simulink library "sensors"  (R2018a)
settings: Solver=VariableStepAuto  StartTime=0.0  StopTime=10.0  RelTol=1e-3
undefined symbols (not defined in the file): magnitude
libraries: simulink_extras x10
settings Model: Creator=David  LastModifiedBy=David

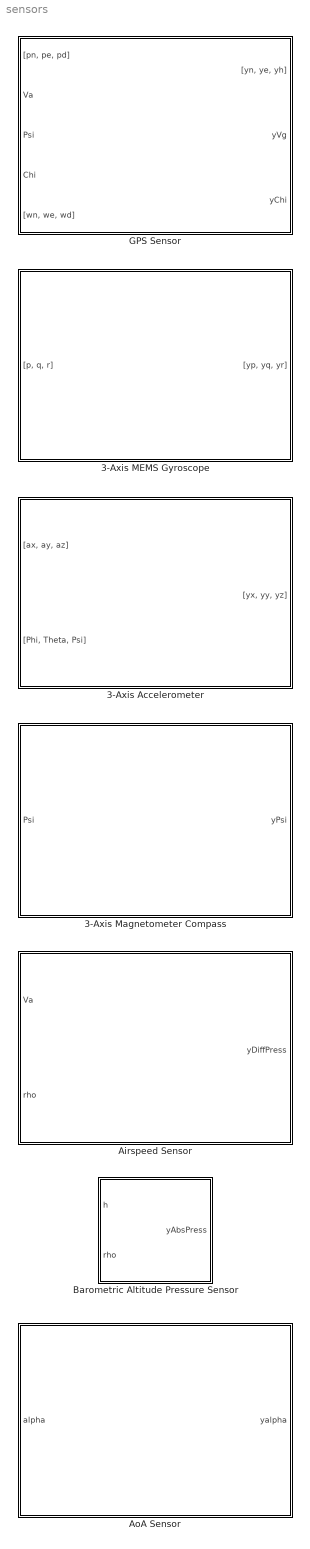
== system sensors ==
  3-Axis Accelerometer : Subsystem  mask{g=9.81, SampleTime=0.01, accelXNoiseDensity=0.1/sqrt(100), accelYNoiseDensity=0.1/sqrt(100), accelZNoiseDensity=0.1/sqrt(100), accelXBandwidthHz=1000, accelYBandwidthHz=1000, accelZBandwidthHz=1000, accelXInit=0, accelYInit=0, accelZInit=0, accelXUpperSaturation=inf, accelXLowerSaturation=-inf, accelYUpperSaturation=inf, accelYLowerSaturation=-inf, accelZUpperSaturation=inf, accelZLowerSaturation=-inf, accelXResolution=1E-12, accelYResolution=1E-12, accelZResolution=1E-12}
      mask prompts: g "Gravity (m/s^2)"; SampleTime "Accelerometer Sample Time (s)"; accelXNoiseDensity "X Accelerometer Noise Density (m/s^2/sqrt(Hz))"; accelYNoiseDensity "Y Accelerometer Noise Density (m/s^2/sqrt(Hz))"; accelZNoiseDensity "Z Accelerometer Noise Density (m/s^2/sqrt(Hz))"; accelXBandwidthHz "X Accelerometer Bandwidth (Hz)"; accelYBandwidthHz "Y Accelerometer Bandwidth (Hz)"; accelZBandwidthHz "Z Accelerometer Bandwidth (Hz)"; accelXInit "X Accelerometer Initial Condition (m/s^2)"; accelYInit "Y Accelerometer Initial Condition (m/s^2)"; accelZInit "Z Accelerometer Initial Condition (m/s^2)"; accelXUpperSaturation "X Accelerometer Measurement Upper Saturation Limit (m/s^2)"; accelXLowerSaturation "X Accelerometer Measurement Lower Saturation Limit (m/s^2)"; accelYUpperSaturation "Y Accelerometer Measurement Upper Saturation Limit (m/s^2)"; accelYLowerSaturation "Y Accelerometer Measurement Lower Saturation Limit (m/s^2)"; accelZUpperSaturation "Z Accelerometer Measurement Upper Saturation Limit (m/s^2)"; accelZLowerSaturation "Z Accelerometer Measurement Upper Saturation Limit (m/s^2)"; accelXResolution "X Accelerometer Resolution (m/s^2)"; accelYResolution "Y Accelerometer Resolution (m/s^2)"; accelZResolution "Z Accelerometer Resolution (m/s^2)"
      mask DialogControl DescGroupVar Prompt: MEMS Accelerometer Model
      mask DialogControl DescTextVar Prompt: MEMS Accelerometer Model with White Noise Modelling
      mask DialogControl Container7 Prompt: System Characteristics
      mask DialogControl Container4 Prompt: Noise Characteristics
      mask DialogControl Container8 Prompt: Density
      mask DialogControl Container10 Prompt: Sensor Dynamics
      mask DialogControl Container13 Prompt: Bandwidth
      mask DialogControl Container12 Prompt: Initial Conditions
      mask DialogControl Container15 Prompt: Limits and Quantization
      mask DialogControl Container17 Prompt: Limits
      mask DialogControl Container20 Prompt: Quantization
      mask DialogControl Control2 Prompt: This can be calculated with the following equation:
      mask DialogControl Control3 Prompt: Physical Resolution = measurement_span/(2^resolution_bits - 1)
      mask Display:
      | image('mems_accel.png')
      | 
      | color('red')
      | 
      | port_label('input', 1, '[a_x, a_y, a_z] (m/s^2)', 'texMode', 'on')
      | port_label('input', 2, '[\phi, \theta, \psi] (rad)', 'texMode', 'on')
      | 
      | port_label('output', 1, '[y_{accel_x}, y_{accel_y}, y_{accel_z}] (m/s^2)', 'texMode', 'on')
  3-Axis MEMS Gyroscope : Subsystem  mask{SampleTime=0.01, gyroXNoiseDensity=0, gyroYNoiseDensity=0, gyroZNoiseDensity=0, gyroXBandwidthHz=1E06, gyroYBandwidthHz=1E06, gyroZBandwidthHz=1E06, gyroXInit=0, gyroYInit=0, gyroZInit=0, gyroXUpperSaturation=inf, gyroXLowerSaturation=-inf, gyroYUpperSaturation=inf, gyroYLowerSaturation=-inf, gyroZUpperSaturation=inf, gyroZLowerSaturation=-inf, gyroXResolution=1E-06, gyroYResolution=1E-06, gyroZResolution=1E-06}
      mask prompts: SampleTime "Gyroscope Sample Time (s)"; gyroXNoiseDensity "X Gyroscope Noise Density (rad/s/sqrt(Hz))"; gyroYNoiseDensity "Y Gyroscope Noise Density (rad/s/sqrt(Hz))"; gyroZNoiseDensity "Z Gyroscope Noise Density (rad/s/sqrt(Hz))"; gyroXBandwidthHz "X Gyroscope Bandwidth (Hz)"; gyroYBandwidthHz "Y Gyroscope Bandwidth (Hz)"; gyroZBandwidthHz "Z Gyroscope Bandwidth (Hz)"; gyroXInit "X Gyroscope Initial Condition (rad/s)"; gyroYInit "Y Gyroscope Initial Condition (rad/s)"; gyroZInit "Z Gyroscope Initial Condition (rad/s)"; gyroXUpperSaturation "X Gyroscope Measurement Upper Saturation Limit (rad/s)"; gyroXLowerSaturation "X Gyroscope Measurement Lower Saturation Limit (rad/s)"; gyroYUpperSaturation "Y Gyroscope Measurement Upper Saturation Limit (rad/s)"; gyroYLowerSaturation "Y Gyroscope Measurement Lower Saturation Limit (rad/s)"; gyroZUpperSaturation "Z Gyroscope Measurement Upper Saturation Limit (rad/s)"; gyroZLowerSaturation "Z Gyroscope Measurement Lower Saturation Limit (rad/s)"; gyroXResolution "X Gyroscope Resolution (rad/s)"; gyroYResolution "Y Gyroscope Resolution (rad/s)"; gyroZResolution "Z Gyroscope Resolution (rad/s)"
      mask DialogControl DescGroupVar Prompt: MEMS Gyroscope Model
      mask DialogControl DescTextVar Prompt: MEMS Gyroscope Model with White Noise Modelling
      mask DialogControl Container7 Prompt: System Characteristics
      mask DialogControl Container4 Prompt: Noise Characteristics
      mask DialogControl Container6 Prompt: Sensor Dynamics
      mask DialogControl Container9 Prompt: Bandwidth
      mask DialogControl Container10 Prompt: Initial Conditions
      mask DialogControl Container11 Prompt: Limits and Quantization
      mask DialogControl Container13 Prompt: Limits
      mask DialogControl Container14 Prompt: Quantization
      mask DialogControl Control3 Prompt: This can be calculated with the following equation:
      mask DialogControl Control2 Prompt: Physical Resolution = measurement_span/(2^resolution_bits - 1)
      mask Display:
      | image('mems_gyro.jpg')
      | 
      | color('red')
      | 
      | port_label('input', 1, '[p, q, r] (rad/s)', 'texMode', 'on')
      | 
      | port_label('output', 1, '[y_{gyro_p}, y_{gyro_q}, y_{gyro_r}] (rad/s)', 'texMode', 'on')
  3-Axis Magnetometer Compass : Subsystem  mask{SampleTime=1, headingNoiseDensity=0, headingBandwidthHz=1E06, headingInit=0, headingUpperSaturation=inf, headingLowerSaturation=-inf, headingResolution=1E-06}
      mask prompts: SampleTime "Magnetometer Sample Time (s)"; headingNoiseDensity "Magnetometer Heading Noise Density (rad/sqrt(Hz))"; headingBandwidthHz "Magnetometer Heading Sensor Bandwidth (Hz)"; headingInit "Magnetometer Heading Sensor Initial Condition (rad)"; headingUpperSaturation "Magnetometer Heading Sensor Upper Saturation Limit (rad)"; headingLowerSaturation "Magnetometer Heading Sensor Lower Saturation Limit (rad)"; headingResolution "Magnetometer Heading Sensor Resolution (rad)"
      mask DialogControl DescGroupVar Prompt: MEMS Magnetometer Model
      mask DialogControl DescTextVar Prompt: MEMS Magnetometer Model to Estimate Heading Angle with White Noise Modelling
      mask DialogControl Container7 Prompt: System Characteristics
      mask DialogControl Container4 Prompt: Noise Characteristics
      mask DialogControl Container6 Prompt: Sensor Dynamics
      mask DialogControl Container10 Prompt: Bandwidth
      mask DialogControl Container11 Prompt: Initial Conditions
      mask DialogControl Container8 Prompt: Limits and Quantization
      mask DialogControl Container13 Prompt: Limits
      mask DialogControl Container14 Prompt: Quantization
      mask Display:
      | image('mems_compass.jpg')
      | 
      | color('red')
      | 
      | port_label('input', 1, '\psi (rad)', 'texMode', 'on')
      | 
      | port_label('output', 1, 'y_{\psi} (rad)', 'texMode', 'on')
  Airspeed Sensor : Subsystem  mask{SampleTime=1, diffPressureStdDev=0, diffPressureBandwidthHz=1E06, diffPressureInit=0, diffPressureUpperSaturation=inf, diffPressureLowerSaturation=-inf, diffPressureResolution=1E-12}
      mask prompts: SampleTime "Airspeed Sensor Sample Time (s)"; diffPressureStdDev "Airspeed Pressure Sensor Noise Std Dev (Pa)"; diffPressureBandwidthHz "Airspeed Pressure Sensor Bandwidth (Hz)"; diffPressureInit "Airspeed Pressure Sensor Initial Condition (Pa)"; diffPressureUpperSaturation "Airspeed Pressure Sensor Upper Saturation Limit (Pa)"; diffPressureLowerSaturation "Airspeed Pressure Sensor Lower Saturation Limit (Pa)"; diffPressureResolution "Airspeed Pressure Sensor Resolution (Pa)"
      mask DialogControl DescGroupVar Prompt: Pitot Tube Airspeed Sensor Model
      mask DialogControl DescTextVar Prompt: Pitot Tube Airspeed Sensor with White Noise Modelling.
      mask DialogControl Control2 Prompt: If one can only get a sensor accuracy of +- error band of span, treat this as 4 sigma when calculating noise density (8 sigma ~ peak-to-peak). (ie. std dev = ((Sensor % Band)/4)*Span )
      mask DialogControl Container7 Prompt: System Characteristics
      mask DialogControl Container4 Prompt: Noise Characteristics
      mask DialogControl Container6 Prompt: Sensor Dynamics
      mask DialogControl Container10 Prompt: Bandwidth
      mask DialogControl Container11 Prompt: Initial Conditions
      mask DialogControl Container8 Prompt: Limits and Quantization
      mask DialogControl Container13 Prompt: Limits
      mask DialogControl Container16 Prompt: Quantization
      mask Display:
      | image('airspeed_sensor.jpg')
      | 
      | color('green')
      | 
      | port_label('input', 1, 'V_a (m/s)', 'texMode', 'on')
      | port_label('input', 2, '\rho (kg/m^3)', 'texMode', 'on')
      | 
      | port_label('output', 1, 'y_{\DeltaP_{V_a}} (Pa)', 'texMode', 'on')
  AoA Sensor : Subsystem  mask{SampleTime=1, alphaStdDev=0, alphaBandwidthHz=1E06, alphaInit=0, alphaUpperSaturation=inf, alphaLowerSaturation=-inf, alphaResolution=1E-12}
      mask prompts: SampleTime "AoA Sensor Sample Time (s)"; alphaStdDev "AoA Sensor Noise Std Dev (rad)"; alphaBandwidthHz "AoA Sensor Bandwidth (Hz)"; alphaInit "AoA Sensor Initial Condition (rad)"; alphaUpperSaturation "AoA Sensor Upper Saturation Limit (rad)"; alphaLowerSaturation "AoA Sensor Lower Saturation Limit (rad)"; alphaResolution "AoA Sensor Resolution (rad)"
      mask DialogControl DescGroupVar Prompt: Pitot Tube Airspeed Sensor Model
      mask DialogControl DescTextVar Prompt: Angle of attack (alpha/AoA) sensor with White Noise Modelling.
      mask DialogControl Container7 Prompt: System Characteristics
      mask DialogControl Container4 Prompt: Noise Characteristics
      mask DialogControl Container6 Prompt: Sensor Dynamics
      mask DialogControl Container10 Prompt: Bandwidth
      mask DialogControl Container11 Prompt: Initial Conditions
      mask DialogControl Container8 Prompt: Limits and Quantization
      mask DialogControl Container13 Prompt: Limits
      mask DialogControl Container16 Prompt: Quantization
      mask Display:
      | image('aoa_sensor.png')
      | 
      | color('green')
      | 
      | port_label('input', 1, '\alpha (rad)', 'texMode', 'on')
      | 
      | port_label('output', 1, 'y_{\alpha} (rad)', 'texMode', 'on')
  Barometric Altitude Pressure Sensor : Subsystem  mask{g=9.81, SampleTime=1, absPressureStdDev=0, absPressureBandwidthHz=1E06, absPressureInit=0, absPressureUpperSaturation=inf, absPressureLowerSaturation=-inf, absPressureResolution=1E-12}
      mask prompts: g "Gravity (m/s^2)"; SampleTime "Barometric Altitude Pressure Sensor Sample Time (s)"; absPressureStdDev "Barometric Altitude Pressure Sensor Noise Std Dev (Pa)"; absPressureBandwidthHz "Barometric Altitude Pressure Sensor Bandwidth (Hz)"; absPressureInit "Barometric Altitude Pressure Sensor Initial Condition (Pa)"; absPressureUpperSaturation "Barometric Altitude Sensor Upper Saturation Limit (Pa)"; absPressureLowerSaturation "Barometric Altitude Sensor Lower Saturation Limit (Pa)"; absPressureResolution "Barometric Altitude Pressure Sensor Resolution (Pa)"
      mask DialogControl DescGroupVar Prompt: Barometric Altitude Pressure Sensor Model
      mask DialogControl DescTextVar Prompt: Barometric Altitude Pressure Sensor with White Noise Modelling.
      mask DialogControl Control2 Prompt: If one can only get a sensor accuracy of +- error band of span, treat this as 4 sigma when calculating noise density (8 sigma ~ peak-to-peak). (ie. std dev = ((Sensor % Band)/4)*Span )
      mask DialogControl Container7 Prompt: System Characteristics
      mask DialogControl Container4 Prompt: Noise Characteristics
      mask DialogControl Container6 Prompt: Sensor Dynamics
      mask DialogControl Container10 Prompt: Bandwidth
      mask DialogControl Container11 Prompt: Initial Conditions
      mask DialogControl Container8 Prompt: Limits and Quantization
      mask DialogControl Container13 Prompt: Limits
      mask DialogControl Container16 Prompt: Quantization
      mask Display:
      | image('barometer.jpg')
      | 
      | color('green')
      | 
      | port_label('input', 1, 'h (m)', 'texMode', 'on')
      | port_label('input', 2, '\rho (kg/m^3)', 'texMode', 'on')
      | 
      | port_label('output', 1, 'y_{P_{abs}} (Pa)', 'texMode', 'on')
  GPS Sensor : Subsystem  mask{SampleTime=0.2, pnInit=0, peInit=0, pdInit=0, VgInit=0, ChiInit=0, GPSNStdDev=0.21, OneOverkGPSN=1100, GPSEStdDev=0.21, OneOverkGPSE=1100, GPSAltStdDev=0.4, OneOverkGPSAlt=1100, GPSVStdDev=0.2}
      mask prompts: SampleTime "GPS Sample Time (s)"; pnInit "Initial North Position (m)"; peInit "Initial East Position (m)"; pdInit "Initial Down Position (m) (-altitude)"; VgInit "Initial Vg (m/s)"; ChiInit "Initial Chi (rad)"; GPSNStdDev "GPS North Std Dev (m)"; OneOverkGPSN "GPS North Time Constant (s)"; GPSEStdDev "GPS East Std Dev (m)"; OneOverkGPSE "GPS East Time Constant (s)"; GPSAltStdDev "GPS Altitude Std Dev (m)"; OneOverkGPSAlt "GPS Altitude Time Constant (s)"; GPSVStdDev "GPS Velocity Std Dev (m/s)"
      mask DialogControl DescGroupVar Prompt: GPS Sensor Model
      mask DialogControl DescTextVar Prompt: GPS Sensor Model Making use of a Gauss-Markov process for noise modelling
      mask DialogControl Container4 Prompt: System Characteristics
      mask DialogControl Container5 Prompt: Noise Characteristics
      mask Display:
      | image('PiksiMulti_GPS.jpg')
      | 
      | color('green')
      | 
      | port_label('input', 1, '[p_N, p_E, p_D] (m)', 'texMode', 'On')
      | port_label('input', 2, 'V_a (m/s)', 'texMode', 'On')
      | port_label('input', 3, '\psi (rad)', 'texMode', 'On')
      | port_label('input', 4, '\chi (rad)', 'texMode', 'On')
      | port_label('input', 5, '[w_N, w_E, w_D] (m/s)', 'texMode', 'On')
      | 
      | port_label('output', 1, '[y_{GPS_N}, y_{GPS_E}, y_{GPS_h}] (m)', 'texMode', 'On')
      | port_label('output', 2, 'y_{GPS_{Vg}} (m/s)', 'texMode', 'On')
      | port_label('output', 3, 'y_{GPS_{\chi}} (rad)', 'texMode', 'On')

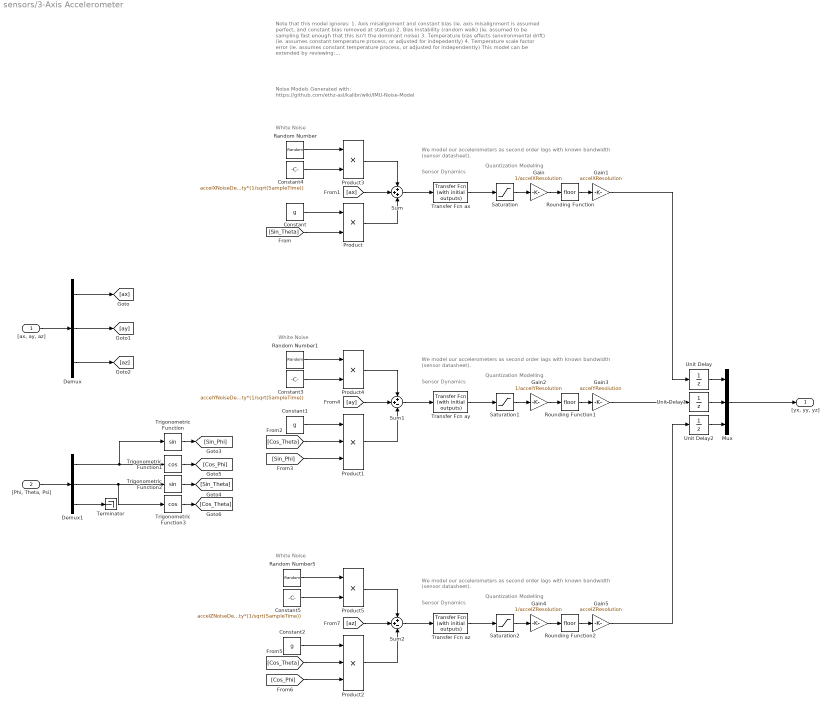
== system sensors/3-Axis Accelerometer ==
  note: Quantization Modelling
  note: Sensor Dynamics
  note: Note that this model ignores:
      | 1. Axis misalignment and constant bias (ie. axis misalignment is assumed perfect, and constant bias removed at startup)
      | 2. Bias Instability (random walk) (ie. assumed to be sampling fast enough that this isn't the dominant noise)
      | 3. Temperature bias effects (environmental drift) (ie. assumes constant temperature process, or adjusted for indepedently)
      | 4. Temperature scale factor error (ie. assumes constant temperature process, or adjusted for independently)
      |
      | This model can be extended by reviewing:
      | https://www.mathworks.com/help/fusion/ref/imusensor-system-object.html?searchHighlight=imuSensor&s_tid=doc_srchtitle
  note: We model our accelerometers as second order lags with known bandwidth
      | (sensor datasheet).
  note: White Noise
  note: Noise Models Generated with:
      | https://github.com/ethz-asl/kalibr/wiki/IMU-Noise-Model
  note: White Noise
  note: White Noise
  note: We model our accelerometers as second order lags with known bandwidth
      | (sensor datasheet).
  note: Quantization Modelling
  note: Sensor Dynamics
  note: We model our accelerometers as second order lags with known bandwidth
      | (sensor datasheet).
  note: Quantization Modelling
  note: Sensor Dynamics
  "[ax, ay, az]" : Inport
  "[Phi, Theta, Psi]" : Inport  Port=2
  Constant : Constant  Value=g
  Constant1 : Constant  Value=g
  Constant2 : Constant  Value=g
  Constant3 : Constant  Value=accelYNoiseDensity*(1/sqrt(SampleTime))
  Constant4 : Constant  Value=accelXNoiseDensity*(1/sqrt(SampleTime))
  Constant5 : Constant  Value=accelZNoiseDensity*(1/sqrt(SampleTime))
  Demux : Demux  Outputs=3
  Demux1 : Demux  Outputs=3
  Gain : Gain  Gain=1/accelXResolution
  Gain1 : Gain  Gain=accelXResolution
  Gain2 : Gain  Gain=1/accelYResolution
  Gain3 : Gain  Gain=accelYResolution
  Gain4 : Gain  Gain=1/accelZResolution
  Gain5 : Gain  Gain=accelZResolution
  Mux : Mux  Inputs=3
  Product{,3..5} (4 alike) : Product
  Product1 : Product  Inputs=3
  Product2 : Product  Inputs=3
  Random Number : RandomNumber  SampleTime=SampleTime
  Random Number1 : RandomNumber  SampleTime=SampleTime
  Random Number5 : RandomNumber  SampleTime=SampleTime
  Rounding Function : Rounding
  Rounding Function1 : Rounding
  Rounding Function2 : Rounding
  Saturation : Saturate  UpperLimit=accelXUpperSaturation  LowerLimit=accelXLowerSaturation  ZeroCross=off
  Saturation1 : Saturate  UpperLimit=accelYUpperSaturation  LowerLimit=accelYLowerSaturation  ZeroCross=off
  Saturation2 : Saturate  UpperLimit=accelZUpperSaturation  LowerLimit=accelZLowerSaturation  ZeroCross=off
  Sum : Sum  Inputs=+++
  Sum1 : Sum  Inputs=++-
  Sum2 : Sum  Inputs=++-
  Terminator : Terminator
  Transfer Fcn ax : simulink_extras/Additional Linear/Transfer Fcn (with initial outputs)  N=[(accelXBandwidthHz*2*pi)^2]  D="[1,  2*accelXBandwidthHz*2*pi, (accelXBandwidthHz*2*pi)^2]"  Y0=accelXInit  U0=accelXInit
  Transfer Fcn ay : simulink_extras/Additional Linear/Transfer Fcn (with initial outputs)  N=[(accelYBandwidthHz*2*pi)^2]  D="[1,  2*accelYBandwidthHz*2*pi, (accelYBandwidthHz*2*pi)^2]"  Y0=accelXInit  U0=accelXInit
  Transfer Fcn az : simulink_extras/Additional Linear/Transfer Fcn (with initial outputs)  N=[(accelZBandwidthHz*2*pi)^2]  D="[1,  2*accelZBandwidthHz*2*pi, (accelZBandwidthHz*2*pi)^2]"  Y0=accelXInit  U0=accelXInit
  Trigonometric Function : Trigonometry
  Trigonometric Function1 : Trigonometry  Operator=cos
  Trigonometric Function2 : Trigonometry
  Trigonometric Function3 : Trigonometry  Operator=cos
  Unit Delay : UnitDelay  InitialCondition=accelXInit  SampleTime=SampleTime
  Unit Delay1 : UnitDelay  InitialCondition=accelYInit  SampleTime=SampleTime
  Unit Delay2 : UnitDelay  InitialCondition=accelZInit  SampleTime=SampleTime
  "[yx, yy, yz]" : Outport
  wires:
  Product/1 -> Sum/3
  [ax] -> Sum/2
  Trigonometric Function3/1 -> [Cos_Theta]
  Sum/1 -> Transfer Fcn ax/1
  Mux/1 -> "[yx, yy, yz]"/1
  [Cos_Phi] -> Product2/3
  Trigonometric Function2/1 -> [Sin_Theta]
  Constant2/1 -> Product2/1
  Demux1/1 -> Trigonometric Function1/1, Trigonometric Function/1
  Demux1/2 -> Trigonometric Function3/1, Trigonometric Function2/1
  [Sin_Theta] -> Product/2
  "[Phi, Theta, Psi]"/1 -> Demux1/1
  [Cos_Theta] -> Product2/2
  [az] -> Sum2/2
  [Cos_Theta] -> Product1/2
  Product2/1 -> Sum2/3
  Trigonometric Function/1 -> [Sin_Phi]
  [ay] -> Sum1/2
  Product1/1 -> Sum1/3
  [Sin_Phi] -> Product1/3
  Trigonometric Function1/1 -> [Cos_Phi]
  Constant1/1 -> Product1/1
  Constant/1 -> Product/1
  Demux1/3 -> Terminator/1
  "[ax, ay, az]"/1 -> Demux/1
  Random Number/1 -> Product3/1
  Constant4/1 -> Product3/2
  Constant3/1 -> Product4/2
  Constant5/1 -> Product5/2
  Demux/1 -> [ax]
  Demux/2 -> [ay]
  Demux/3 -> [az]
  Product3/1 -> Sum/1
  Product4/1 -> Sum1/1
  Random Number1/1 -> Product4/1
  Random Number5/1 -> Product5/1
  Product5/1 -> Sum2/1
  Saturation/1 -> Gain/1
  Transfer Fcn ax/1 -> Saturation/1
  Gain/1 -> Rounding Function/1
  Rounding Function/1 -> Gain1/1
  Gain1/1 -> Unit Delay/1
  Gain2/1 -> Rounding Function1/1
  Saturation1/1 -> Gain2/1
  Transfer Fcn ay/1 -> Saturation1/1
  Rounding Function1/1 -> Gain3/1
  Sum1/1 -> Transfer Fcn ay/1
  Gain3/1 -> Unit Delay1/1
  Gain5/1 -> Unit Delay2/1
  Sum2/1 -> Transfer Fcn az/1
  Rounding Function2/1 -> Gain5/1
  Saturation2/1 -> Gain4/1
  Transfer Fcn az/1 -> Saturation2/1
  Gain4/1 -> Rounding Function2/1
  Unit Delay/1 -> Mux/1
  Unit Delay1/1 -> Mux/2
  Unit Delay2/1 -> Mux/3

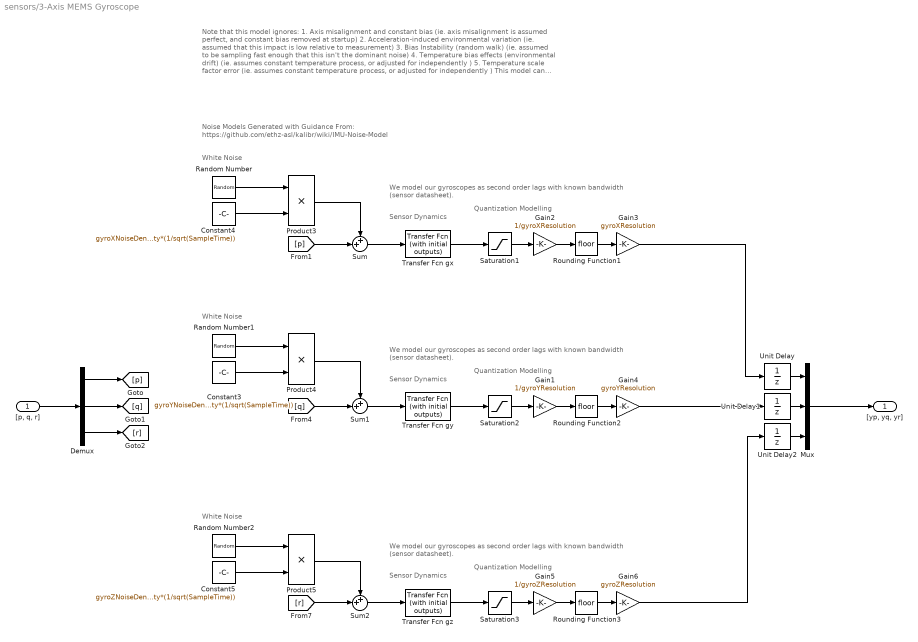
== system sensors/3-Axis MEMS Gyroscope ==
  note: White Noise
  note: Noise Models Generated with Guidance From:
      | https://github.com/ethz-asl/kalibr/wiki/IMU-Noise-Model
  note: White Noise
  note: White Noise
  note: We model our gyroscopes as second order lags with known bandwidth
      | (sensor datasheet).
  note: Quantization Modelling
  note: Sensor Dynamics
  note: Quantization Modelling
  note: Sensor Dynamics
  note: We model our gyroscopes as second order lags with known bandwidth
      | (sensor datasheet).
  note: Quantization Modelling
  note: We model our gyroscopes as second order lags with known bandwidth
      | (sensor datasheet).
  note: Sensor Dynamics
  note: Note that this model ignores:
      | 1. Axis misalignment and constant bias (ie. axis misalignment is assumed perfect, and constant bias removed at startup)
      | 2. Acceleration-induced environmental variation (ie. assumed that this impact is low relative to measurement)
      | 3. Bias Instability (random walk) (ie. assumed to be sampling fast enough that this isn't the dominant noise)
      | 4. Temperature bias effects (environmental drift) (ie. assumes constant temperature process, or adjusted for independently )
      | 5. Temperature scale factor error (ie. assumes constant temperature process, or adjusted for independently )
      |
      | This model can be extended by reviewing:
      | https://www.mathworks.com/help/fusion/ref/imusensor-system-object.html?searchHighlight=imuSensor&s_tid=doc_srchtitle
  "[p, q, r]" : Inport
  Constant3 : Constant  Value=gyroYNoiseDensity*(1/sqrt(SampleTime))
  Constant4 : Constant  Value=gyroXNoiseDensity*(1/sqrt(SampleTime))
  Constant5 : Constant  Value=gyroZNoiseDensity*(1/sqrt(SampleTime))
  Demux : Demux  Outputs=3
  Gain1 : Gain  Gain=1/gyroYResolution
  Gain2 : Gain  Gain=1/gyroXResolution
  Gain3 : Gain  Gain=gyroXResolution
  Gain4 : Gain  Gain=gyroYResolution
  Gain5 : Gain  Gain=1/gyroZResolution
  Gain6 : Gain  Gain=gyroZResolution
  Mux : Mux  Inputs=3
  Product3 : Product
  Product4 : Product
  Product5 : Product
  Random Number : RandomNumber  SampleTime=SampleTime
  Random Number1 : RandomNumber  SampleTime=SampleTime
  Random Number2 : RandomNumber  SampleTime=SampleTime
  Rounding Function1 : Rounding
  Rounding Function2 : Rounding
  Rounding Function3 : Rounding
  Saturation1 : Saturate  UpperLimit=gyroXUpperSaturation  LowerLimit=gyroXLowerSaturation
  Saturation2 : Saturate  UpperLimit=gyroYUpperSaturation  LowerLimit=gyroYLowerSaturation
  Saturation3 : Saturate  UpperLimit=gyroZUpperSaturation  LowerLimit=gyroZLowerSaturation
  Sum : Sum  Inputs=++|
  Sum1 : Sum  Inputs=++|
  Sum2 : Sum  Inputs=++|
  Transfer Fcn gx : simulink_extras/Additional Linear/Transfer Fcn (with initial outputs)  N=[(gyroXBandwidthHz*2*pi)^2]  D="[1,  2*gyroXBandwidthHz*2*pi, (gyroXBandwidthHz*2*pi)^2]"  Y0=gyroXInit  U0=gyroXInit
  Transfer Fcn gy : simulink_extras/Additional Linear/Transfer Fcn (with initial outputs)  N=[(gyroYBandwidthHz*2*pi)^2]  D="[1,  2*gyroYBandwidthHz*2*pi, (gyroYBandwidthHz*2*pi)^2]"  Y0=gyroYInit  U0=gyroYInit
  Transfer Fcn gz : simulink_extras/Additional Linear/Transfer Fcn (with initial outputs)  N=[(gyroZBandwidthHz*2*pi)^2]  D="[1,  2*gyroZBandwidthHz*2*pi, (gyroZBandwidthHz*2*pi)^2]"  Y0=gyroZInit  U0=gyroZInit
  Unit Delay : UnitDelay  InitialCondition=gyroXInit  SampleTime=SampleTime
  Unit Delay1 : UnitDelay  InitialCondition=gyroYInit  SampleTime=SampleTime
  Unit Delay2 : UnitDelay  InitialCondition=gyroZInit  SampleTime=SampleTime
  "[yp, yq, yr]" : Outport
  wires:
  [p] -> Sum/2
  Demux/3 -> [r]
  Mux/1 -> "[yp, yq, yr]"/1
  [r] -> Sum2/2
  [q] -> Sum1/2
  Demux/1 -> [p]
  Demux/2 -> [q]
  "[p, q, r]"/1 -> Demux/1
  Random Number/1 -> Product3/1
  Product3/1 -> Sum/1
  Constant4/1 -> Product3/2
  Random Number1/1 -> Product4/1
  Constant3/1 -> Product4/2
  Product4/1 -> Sum1/1
  Product5/1 -> Sum2/1
  Constant5/1 -> Product5/2
  Random Number2/1 -> Product5/1
  Gain3/1 -> Unit Delay/1
  Sum/1 -> Transfer Fcn gx/1
  Rounding Function1/1 -> Gain3/1
  Saturation1/1 -> Gain2/1
  Transfer Fcn gx/1 -> Saturation1/1
  Gain2/1 -> Rounding Function1/1
  Saturation2/1 -> Gain1/1
  Sum1/1 -> Transfer Fcn gy/1
  Gain4/1 -> Unit Delay1/1
  Rounding Function2/1 -> Gain4/1
  Gain1/1 -> Rounding Function2/1
  Transfer Fcn gy/1 -> Saturation2/1
  Sum2/1 -> Transfer Fcn gz/1
  Gain5/1 -> Rounding Function3/1
  Rounding Function3/1 -> Gain6/1
  Transfer Fcn gz/1 -> Saturation3/1
  Saturation3/1 -> Gain5/1
  Gain6/1 -> Unit Delay2/1
  Unit Delay/1 -> Mux/1
  Unit Delay1/1 -> Mux/2
  Unit Delay2/1 -> Mux/3

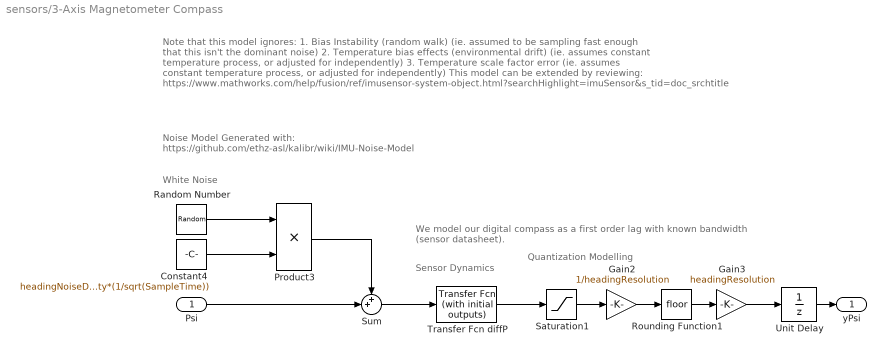
== system sensors/3-Axis Magnetometer Compass ==
  note: White Noise
  note: Noise Model Generated with:
      | https://github.com/ethz-asl/kalibr/wiki/IMU-Noise-Model
  note: Quantization Modelling
  note: We model our digital compass as a first order lag with known bandwidth
      | (sensor datasheet).
  note: Sensor Dynamics
  note: Note that this model ignores:
      | 1. Bias Instability (random walk) (ie. assumed to be sampling fast enough that this isn't the dominant noise)
      | 2. Temperature bias effects (environmental drift) (ie. assumes constant temperature process, or adjusted for independently)
      | 3. Temperature scale factor error (ie. assumes constant temperature process, or adjusted for independently)
      |
      | This model can be extended by reviewing:
      | https://www.mathworks.com/help/fusion/ref/imusensor-system-object.html?searchHighlight=imuSensor&s_tid=doc_srchtitle
  Psi : Inport
  Constant4 : Constant  Value=headingNoiseDensity*(1/sqrt(SampleTime))
  Gain2 : Gain  Gain=1/headingResolution
  Gain3 : Gain  Gain=headingResolution
  Product3 : Product
  Random Number : RandomNumber  SampleTime=SampleTime
  Rounding Function1 : Rounding
  Saturation1 : Saturate  UpperLimit=headingUpperSaturation  LowerLimit=headingLowerSaturation
  Sum : Sum  Inputs=++|
  Transfer Fcn diffP : simulink_extras/Additional Linear/Transfer Fcn (with initial outputs)  N=[headingBandwidthHz*2*pi]  D="[1,  headingBandwidthHz*2*pi]"  Y0=headingInit  U0=headingInit
  Unit Delay : UnitDelay  InitialCondition=headingInit  SampleTime=SampleTime
  yPsi : Outport
  wires:
  Psi/1 -> Sum/2
  Random Number/1 -> Product3/1
  Product3/1 -> Sum/1
  Constant4/1 -> Product3/2
  Sum/1 -> Transfer Fcn diffP/1
  Rounding Function1/1 -> Gain3/1
  Gain2/1 -> Rounding Function1/1
  Saturation1/1 -> Gain2/1
  Transfer Fcn diffP/1 -> Saturation1/1
  Gain3/1 -> Unit Delay/1
  Unit Delay/1 -> yPsi/1

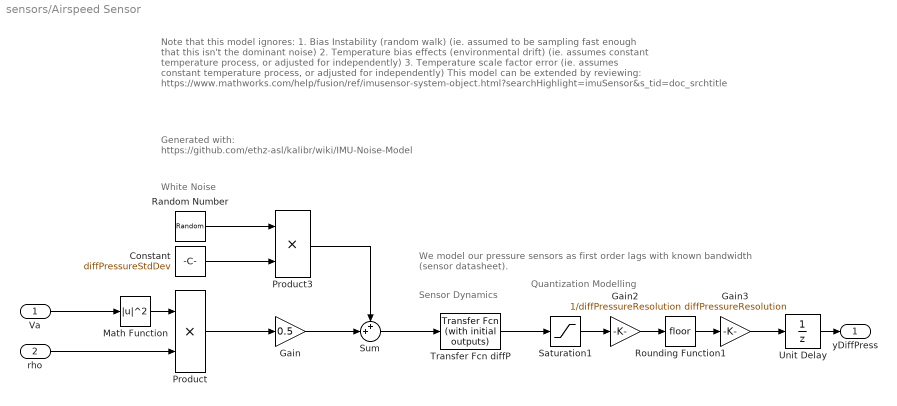
== system sensors/Airspeed Sensor ==
  note: White Noise
  note: Generated with:
      | https://github.com/ethz-asl/kalibr/wiki/IMU-Noise-Model
  note: We model our pressure sensors as first order lags with known bandwidth
      | (sensor datasheet).
  note: Sensor Dynamics
  note: Quantization Modelling
  note: Note that this model ignores:
      | 1. Bias Instability (random walk) (ie. assumed to be sampling fast enough that this isn't the dominant noise)
      | 2. Temperature bias effects (environmental drift) (ie. assumes constant temperature process, or adjusted for independently)
      | 3. Temperature scale factor error (ie. assumes constant temperature process, or adjusted for independently)
      |
      | This model can be extended by reviewing:
      | https://www.mathworks.com/help/fusion/ref/imusensor-system-object.html?searchHighlight=imuSensor&s_tid=doc_srchtitle
  Va : Inport
  rho : Inport  Port=2
  Constant : Constant  Value=diffPressureStdDev
  Gain : Gain  Gain=0.5
  Gain2 : Gain  Gain=1/diffPressureResolution
  Gain3 : Gain  Gain=diffPressureResolution
  Math Function : Math  Operator=magnitude^2  SaturateOnIntegerOverflow=on
  Product : Product
  Product3 : Product
  Random Number : RandomNumber  SampleTime=SampleTime
  Rounding Function1 : Rounding
  Saturation1 : Saturate  UpperLimit=diffPressureUpperSaturation  LowerLimit=diffPressureLowerSaturation
  Sum : Sum  Inputs=++|
  Transfer Fcn diffP : simulink_extras/Additional Linear/Transfer Fcn (with initial outputs)  N=[diffPressureBandwidthHz*2*pi]  D="[1,  diffPressureBandwidthHz*2*pi]"  Y0=diffPressureInit  U0=diffPressureInit
  Unit Delay : UnitDelay  InitialCondition=diffPressureInit  SampleTime=SampleTime
  yDiffPress : Outport
  wires:
  Va/1 -> Math Function/1
  Random Number/1 -> Product3/1
  Product3/1 -> Sum/1
  Constant/1 -> Product3/2
  Math Function/1 -> Product/1
  rho/1 -> Product/2
  Product/1 -> Gain/1
  Gain/1 -> Sum/2
  Transfer Fcn diffP/1 -> Saturation1/1
  Sum/1 -> Transfer Fcn diffP/1
  Gain2/1 -> Rounding Function1/1
  Saturation1/1 -> Gain2/1
  Gain3/1 -> Unit Delay/1
  Rounding Function1/1 -> Gain3/1
  Unit Delay/1 -> yDiffPress/1

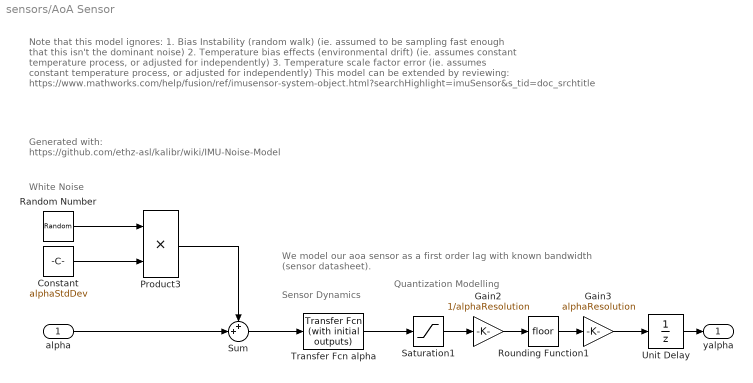
== system sensors/AoA Sensor ==
  note: White Noise
  note: Generated with:
      | https://github.com/ethz-asl/kalibr/wiki/IMU-Noise-Model
  note: We model our aoa sensor as a first order lag with known bandwidth
      | (sensor datasheet).
  note: Sensor Dynamics
  note: Quantization Modelling
  note: Note that this model ignores:
      | 1. Bias Instability (random walk) (ie. assumed to be sampling fast enough that this isn't the dominant noise)
      | 2. Temperature bias effects (environmental drift) (ie. assumes constant temperature process, or adjusted for independently)
      | 3. Temperature scale factor error (ie. assumes constant temperature process, or adjusted for independently)
      |
      | This model can be extended by reviewing:
      | https://www.mathworks.com/help/fusion/ref/imusensor-system-object.html?searchHighlight=imuSensor&s_tid=doc_srchtitle
  alpha : Inport
  Constant : Constant  Value=alphaStdDev
  Gain2 : Gain  Gain=1/alphaResolution
  Gain3 : Gain  Gain=alphaResolution
  Product3 : Product
  Random Number : RandomNumber  SampleTime=SampleTime
  Rounding Function1 : Rounding
  Saturation1 : Saturate  UpperLimit=alphaUpperSaturation  LowerLimit=alphaLowerSaturation
  Sum : Sum  Inputs=++|
  Transfer Fcn alpha : simulink_extras/Additional Linear/Transfer Fcn (with initial outputs)  N=[alphaBandwidthHz*2*pi]  D="[1,  alphaBandwidthHz*2*pi]"  Y0=alphaInit  U0=alphaInit
  Unit Delay : UnitDelay  InitialCondition=alphaInit  SampleTime=SampleTime
  yalpha : Outport
  wires:
  Random Number/1 -> Product3/1
  Product3/1 -> Sum/1
  Constant/1 -> Product3/2
  alpha/1 -> Sum/2
  Transfer Fcn alpha/1 -> Saturation1/1
  Sum/1 -> Transfer Fcn alpha/1
  Gain2/1 -> Rounding Function1/1
  Saturation1/1 -> Gain2/1
  Gain3/1 -> Unit Delay/1
  Rounding Function1/1 -> Gain3/1
  Unit Delay/1 -> yalpha/1

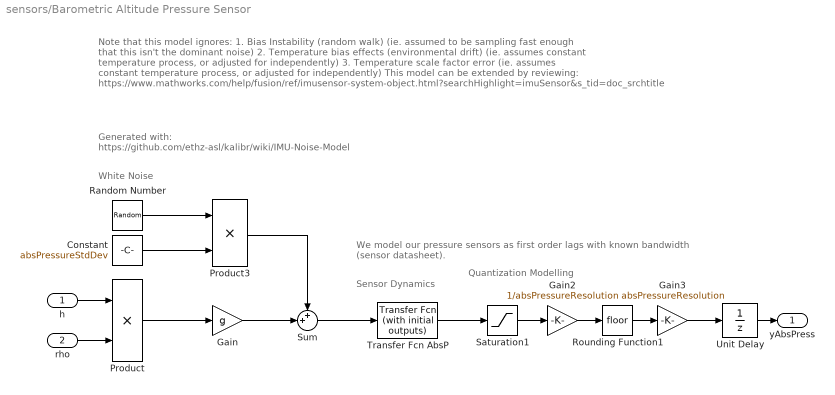
== system sensors/Barometric Altitude Pressure Sensor ==
  note: Generated with:
      | https://github.com/ethz-asl/kalibr/wiki/IMU-Noise-Model
  note: We model our pressure sensors as first order lags with known bandwidth
      | (sensor datasheet).
  note: Sensor Dynamics
  note: Quantization Modelling
  note: Note that this model ignores:
      | 1. Bias Instability (random walk) (ie. assumed to be sampling fast enough that this isn't the dominant noise)
      | 2. Temperature bias effects (environmental drift) (ie. assumes constant temperature process, or adjusted for independently)
      | 3. Temperature scale factor error (ie. assumes constant temperature process, or adjusted for independently)
      |
      | This model can be extended by reviewing:
      | https://www.mathworks.com/help/fusion/ref/imusensor-system-object.html?searchHighlight=imuSensor&s_tid=doc_srchtitle
  note: White Noise
  h : Inport
  rho : Inport  Port=2
  Constant : Constant  Value=absPressureStdDev
  Gain : Gain  Gain=g
  Gain2 : Gain  Gain=1/absPressureResolution
  Gain3 : Gain  Gain=absPressureResolution
  Product : Product
  Product3 : Product
  Random Number : RandomNumber  SampleTime=SampleTime
  Rounding Function1 : Rounding
  Saturation1 : Saturate  UpperLimit=absPressureUpperSaturation  LowerLimit=absPressureLowerSaturation
  Sum : Sum  Inputs=++|
  Transfer Fcn AbsP : simulink_extras/Additional Linear/Transfer Fcn (with initial outputs)  N=[absPressureBandwidthHz*2*pi]  D="[1,  absPressureBandwidthHz*2*pi]"  Y0=absPressureInit  U0=absPressureInit
  Unit Delay : UnitDelay  InitialCondition=absPressureInit  SampleTime=SampleTime
  yAbsPress : Outport
  wires:
  Transfer Fcn AbsP/1 -> Saturation1/1
  Sum/1 -> Transfer Fcn AbsP/1
  Gain2/1 -> Rounding Function1/1
  Saturation1/1 -> Gain2/1
  Gain3/1 -> Unit Delay/1
  Rounding Function1/1 -> Gain3/1
  Gain/1 -> Sum/2
  Constant/1 -> Product3/2
  Product3/1 -> Sum/1
  Product/1 -> Gain/1
  Random Number/1 -> Product3/1
  rho/1 -> Product/2
  h/1 -> Product/1
  Unit Delay/1 -> yAbsPress/1

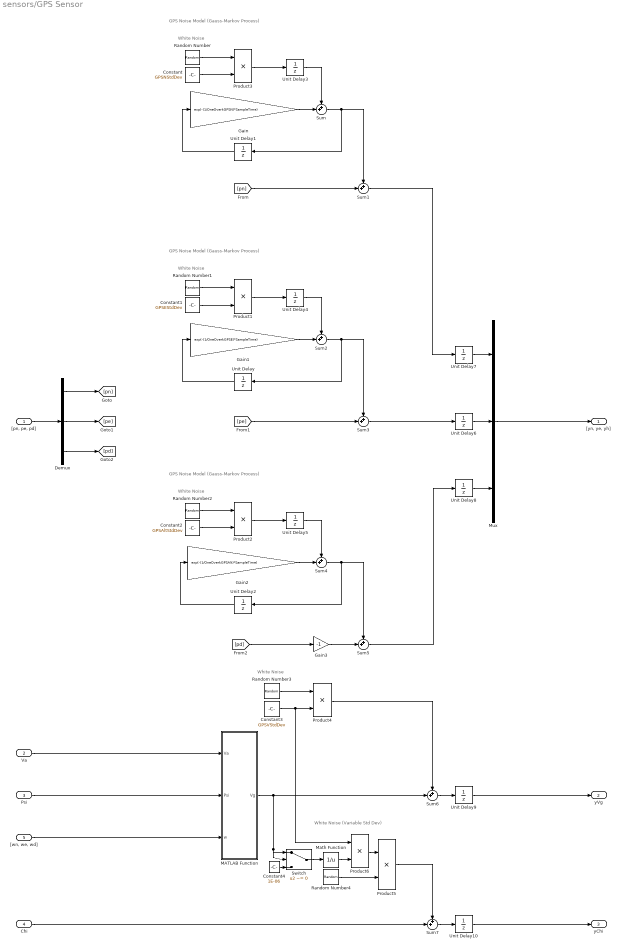
== system sensors/GPS Sensor ==
  note: GPS Noise Model (Gauss-Markov Process)
  note: White Noise
  note: White Noise
  note: GPS Noise Model (Gauss-Markov Process)
  note: White Noise
  note: GPS Noise Model (Gauss-Markov Process)
  note: White Noise
  note: White Noise (Variable Std Dev)
  "[pn, pe, pd]" : Inport
  Va : Inport  Port=2
  Psi : Inport  Port=3
  Chi : Inport  Port=4
  "[wn, we, wd]" : Inport  Port=5
  Constant : Constant  Value=GPSNStdDev
  Constant1 : Constant  Value=GPSEStdDev
  Constant2 : Constant  Value=GPSAltStdDev
  Constant3 : Constant  Value=GPSVStdDev
  Constant4 : Constant  Value=1E-06
  Demux : Demux  Outputs=3
  Gain : Gain  Gain=exp(-(1/OneOverkGPSN)*SampleTime)
  Gain1 : Gain  Gain=exp(-(1/OneOverkGPSE)*SampleTime)
  Gain2 : Gain  Gain=exp(-(1/OneOverkGPSAlt)*SampleTime)
  Gain3 : Gain  Gain=-1
  MATLAB Function : MATLAB Function  TreatAsAtomicUnit=on
  Math Function : Math  Operator=reciprocal  SaturateOnIntegerOverflow=on
  Mux : Mux  Inputs=3
  Product{1..6} (6 alike) : Product
  Random Number{,1..4} (5 alike) : RandomNumber  SampleTime=SampleTime
  Sum{,1..7} (8 alike) : Sum  Inputs=++|
  Switch : Switch  Criteria=u2 ~= 0
  Unit Delay{,1..5} (6 alike) : UnitDelay  SampleTime=SampleTime
  Unit Delay10 : UnitDelay  InitialCondition=ChiInit  SampleTime=SampleTime
  Unit Delay6 : UnitDelay  InitialCondition=peInit  SampleTime=SampleTime
  Unit Delay7 : UnitDelay  InitialCondition=pnInit  SampleTime=SampleTime
  Unit Delay8 : UnitDelay  InitialCondition=pdInit  SampleTime=SampleTime
  Unit Delay9 : UnitDelay  InitialCondition=VgInit  SampleTime=SampleTime
  "[yn, ye, yh]" : Outport
  yVg : Outport  Port=2
  yChi : Outport  Port=3
  wires:
  Constant1/1 -> Product1/2
  [pe] -> Sum3/2
  Gain1/1 -> Sum2/2
  Unit Delay1/1 -> Gain/1
  Sum/1 -> Unit Delay1/1, Sum1/1
  Demux/3 -> [pd]
  Constant/1 -> Product3/2
  Sum2/1 -> Unit Delay/1, Sum3/1
  Unit Delay2/1 -> Gain2/1
  Constant2/1 -> Product2/2
  Sum4/1 -> Unit Delay2/1, Sum5/1
  Unit Delay/1 -> Gain1/1
  Sum3/1 -> Unit Delay6/1
  Random Number/1 -> Product3/1
  Random Number1/1 -> Product1/1
  Gain/1 -> Sum/2
  Sum1/1 -> Unit Delay7/1
  [pn] -> Sum1/2
  Mux/1 -> "[yn, ye, yh]"/1
  Gain2/1 -> Sum4/2
  Random Number2/1 -> Product2/1
  Demux/2 -> [pe]
  Sum5/1 -> Unit Delay8/1
  [pd] -> Gain3/1
  Gain3/1 -> Sum5/2
  "[pn, pe, pd]"/1 -> Demux/1
  Demux/1 -> [pn]
  Product2/1 -> Unit Delay5/1
  Product1/1 -> Unit Delay4/1
  Product3/1 -> Unit Delay3/1
  Unit Delay3/1 -> Sum/1
  Unit Delay4/1 -> Sum2/1
  Unit Delay5/1 -> Sum4/1
  Va/1 -> MATLAB Function/1(Va)
  Constant3/1 -> Product6/1, Product4/2
  Random Number3/1 -> Product4/1
  Product4/1 -> Sum6/1
  MATLAB Function/1(Vg) -> Sum6/2, Switch/1, Switch/2
  Random Number4/1 -> Product5/2
  Sum6/1 -> Unit Delay9/1
  Sum7/1 -> Unit Delay10/1
  Math Function/1 -> Product6/2
  Product6/1 -> Product5/1
  Product5/1 -> Sum7/1
  Chi/1 -> Sum7/2
  Switch/1 -> Math Function/1
  Constant4/1 -> Switch/3
  Psi/1 -> MATLAB Function/2(Psi)
  "[wn, we, wd]"/1 -> MATLAB Function/3(w)
  Unit Delay6/1 -> Mux/2
  Unit Delay7/1 -> Mux/1
  Unit Delay8/1 -> Mux/3
  Unit Delay9/1 -> yVg/1
  Unit Delay10/1 -> yChi/1

== matlab function sensors/GPS Sensor/MATLAB Function ==
  data: Va input size=1; Psi input size=1; Vg output size=1; w input size=3
function Vg = fcn(Va, Psi, w)

    wn = w(1);
    we = w(2);

    Vg = sqrt( (Va*cos(Psi) + wn)^2 + (Va*sin(Psi) + we)^2 );
